simulink model "heaterWithPIController"  (R2020b)
settings: Solver=VariableStepAuto  StartTime=0.0  StopTime=9000  RelTol=1e-3
settings Model: Creator=avi  LastModifiedBy=avi

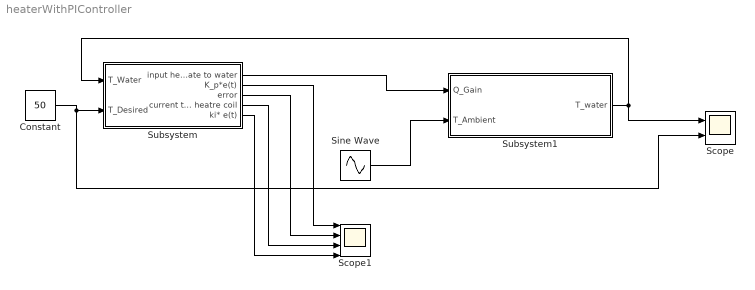
== system heaterWithPIController ==
  Constant : Constant  Value=50
  Scope : Scope  NumInputPorts=2
  Scope1 : Scope  NumInputPorts=4
  Sine Wave : Sin  Amplitude=10  Bias=25  Frequency=.00005  SampleTime=0
  Subsystem : Subsystem
  Subsystem1 : Subsystem
  wires:
  Subsystem1/1(T_water) -> Scope/1, Subsystem/1(T_Water)
  Sine Wave/1 -> Subsystem1/2(T_Ambient)
  Subsystem/1(input heat rate to water) -> Subsystem1/1(Q_Gain)
  Constant/1 -> Scope/2, Subsystem/2(T_Desired)
  Subsystem/2(K_p*e(t)) -> Scope1/1
  Subsystem/4(current to heatre coil) -> Scope1/3
  Subsystem/3(error) -> Scope1/2
  Subsystem/5(ki* e(t)) -> Scope1/4

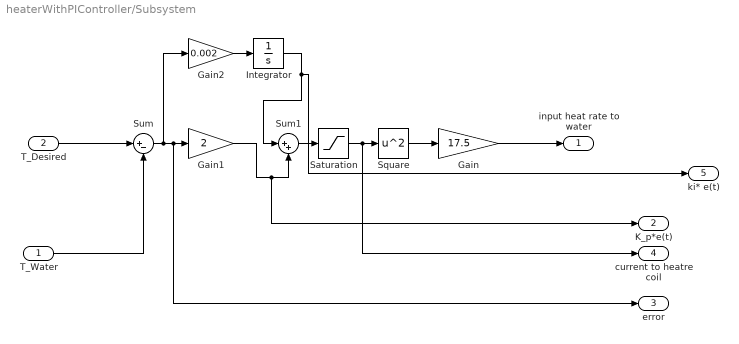
== system heaterWithPIController/Subsystem ==
  T_Water : Inport
  T_Desired : Inport  Port=2
  Gain : Gain  Gain=17.5
  Gain1 : Gain  Gain=2
  Gain2 : Gain  Gain=0.002
  Integrator : Integrator
  Saturation : Saturate  UpperLimit=15  LowerLimit=0
  Square : Math  Operator=square  SaturateOnIntegerOverflow=on
  Sum : Sum  Inputs=|+-
  Sum1 : Sum  Inputs=|++
  input heat rate to water : Outport
  K_p*e(t) : Outport  Port=2
  error : Outport  Port=3
  current to heatre coil : Outport  Port=4
  ki* e(t) : Outport  Port=5
  wires:
  Saturation/1 -> current to heatre coil/1, Square/1
  Sum/1 -> Gain2/1, error/1, Gain1/1
  T_Desired/1 -> Sum/1
  T_Water/1 -> Sum/2
  Gain/1 -> input heat rate to water/1
  Square/1 -> Gain/1
  Sum1/1 -> Saturation/1
  Gain1/1 -> K_p*e(t)/1, Sum1/2
  Gain2/1 -> Integrator/1
  Integrator/1 -> ki* e(t)/1, Sum1/1

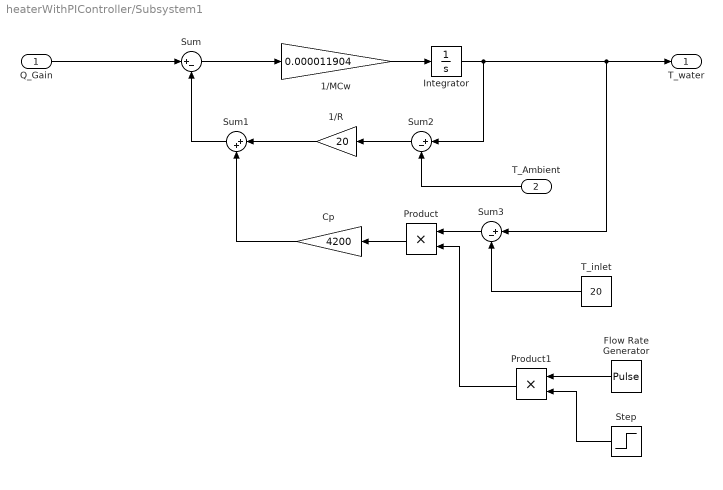
== system heaterWithPIController/Subsystem1 ==
  Q_Gain : Inport
  T_Ambient : Inport  Port=2
  1/MCw : Gain  Gain=0.000011904
  1/R : Gain  Gain=20
  Cp : Gain  Gain=4200
  Flow Rate Generator : DiscretePulseGenerator  PulseType=Time based  Amplitude=7.48/60  Period=300  PulseWidth=50  PhaseDelay=2500
  Integrator : Integrator  InitialCondition=20
  Product : Product
  Product1 : Product
  Step : Step  Time=2500  SampleTime=0
  Sum : Sum  Inputs=|+-
  Sum1 : Sum  Inputs=|++
  Sum2 : Sum  Inputs=|+-
  Sum3 : Sum  Inputs=|+-
  T_inlet : Constant  Value=20
  T_water : Outport
  wires:
  Sum2/1 -> 1/R/1
  Sum3/1 -> Product/1
  1/R/1 -> Sum1/1
  Cp/1 -> Sum1/2
  Flow Rate Generator/1 -> Product1/1
  1/MCw/1 -> Integrator/1
  Sum/1 -> 1/MCw/1
  T_inlet/1 -> Sum3/2
  Sum1/1 -> Sum/2
  Product/1 -> Cp/1
  Integrator/1 -> Sum2/1, T_water/1, Sum3/1
  T_Ambient/1 -> Sum2/2
  Product1/1 -> Product/2
  Step/1 -> Product1/2
  Q_Gain/1 -> Sum/1
